simulink model "test"  (R2021a)
settings: Solver=FixedStepAuto  StartTime=0.0  StopTime=10.0  FixedStep=0.05  RelTol=1e-3
InitFcn:
  | port = 19999;
  | InitSim;
undefined symbols (not defined in the file): clientID, vrep
settings Model: Creator=Harry  LastModifiedBy=Harry

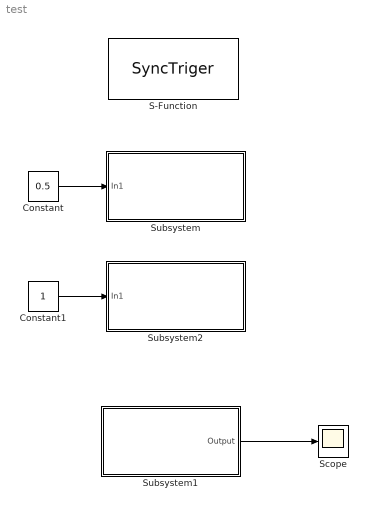
== system test ==
  Constant : Constant  Value=0.5
  Constant1 : Constant
  S-Function : S-Function  FunctionName=SyncTriger  Parameters=vrep,clientID  SFunctionDeploymentMode=off  EnableBusSupport=off
      mask Display:
      | disp('Sync triger');
      | 
      | 
      | color('red')
      | text(5,8,'VrepSim V0.1')
  Scope : Scope
  Subsystem : Subsystem  mask{joint_name='Revolute_joint1', is_use_radian=on}
      mask prompts: joint_name "Joint name"; is_use_radian "Is use radian"
      mask DialogControl DescGroupVar Prompt: Instructions
      mask DialogControl DescTextVar Prompt: ......
      mask Display:
      | if ischar(joint_name)
      |     color('black');
      |     x=sprintf('SetJointVelocity\n%s',joint_name);
      |     disp(x);
      | else
      |     color('red');
      |     disp('Input Error');
      | end
  Subsystem1 : Subsystem  mask{joint_name='Revolute_joint1', is_use_radian=off}
      mask prompts: joint_name "Joint name"; is_use_radian "Is use radian"
      mask DialogControl DescGroupVar Prompt: Instructions
      mask DialogControl DescTextVar Prompt: ......
      mask Display:
      | if ischar(joint_name)
      |     color('black');
      |     x=sprintf('GetJointPosition\n%s',joint_name);
      |     disp(x);
      | else
      |     color('red');
      |     disp('Input Error');
      | end
  Subsystem2 : Subsystem  mask{joint_name='Revolute_joint2', is_use_radian=on}
      mask prompts: joint_name "Joint name"; is_use_radian "Is use radian"
      mask DialogControl DescGroupVar Prompt: Instructions
      mask DialogControl DescTextVar Prompt: ......
      mask Display:
      | if ischar(joint_name)
      |     color('black');
      |     x=sprintf('SetJointVelocity\n%s',joint_name);
      |     disp(x);
      | else
      |     color('red');
      |     disp('Input Error');
      | end
  wires:
  Constant/1 -> Subsystem/1(In1)
  Subsystem1/1(Output) -> Scope/1
  Constant1/1 -> Subsystem2/1(In1)

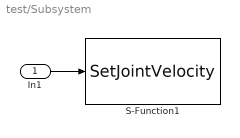
== system test/Subsystem ==
  In1 : Inport
  S-Function1 : S-Function  FunctionName=SetJointVelocity  Parameters=vrep,clientID,joint_name,is_use_radian  SFunctionDeploymentMode=off  EnableBusSupport=off
  wires:
  In1/1 -> S-Function1/1

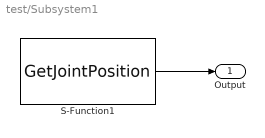
== system test/Subsystem1 ==
  S-Function1 : S-Function  FunctionName=GetJointPosition  Parameters=vrep,clientID,joint_name,is_use_radian  SFunctionDeploymentMode=off  EnableBusSupport=off
  Output : Outport
  wires:
  S-Function1/1 -> Output/1

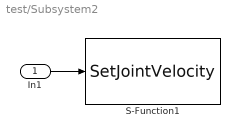
== system test/Subsystem2 ==
  In1 : Inport
  S-Function1 : S-Function  FunctionName=SetJointVelocity  Parameters=vrep,clientID,joint_name,is_use_radian  SFunctionDeploymentMode=off  EnableBusSupport=off
  wires:
  In1/1 -> S-Function1/1
